simulink model "util_quat_hrn"  (R2014b)
settings: Solver=FixedStepDiscrete  StartTime=0.0  StopTime=12  FixedStep=1  RelTol=1e-3
libraries: util_quat_lib x8
settings Model: RequirementInfo={'other' './util_quat_req.html' '' 'true' ' Requirements for Quaternions' '' } %GIDa_d58dfe71_7bd5_46f6_9629_ed2cd7b47ed5  ExtModeAutoUpdateStatusClock=off  Creator=hcannon  LastModifiedBy=mstewart
settings DataIOCC: SignalLoggingSaveFormat=ModelDataLogs
settings OptimizationCC: ExpressionDepthLimit=2147483647  InitFltsAndDblsToZero=on
settings DebuggingCC: UnderspecifiedInitializationDetection=Classic  MergeDetectMultiDrivingBlocksExec=none  FcnCallInpInsideContextMsg=UseLocalSettings  StateNameClashWarn=warning  StrictBusMsg=Warning
settings SFSimCC: SimParseCustomCode=off
settings GRTTargetCC: CombineOutputUpdateFcns=off  GRTInterface=on

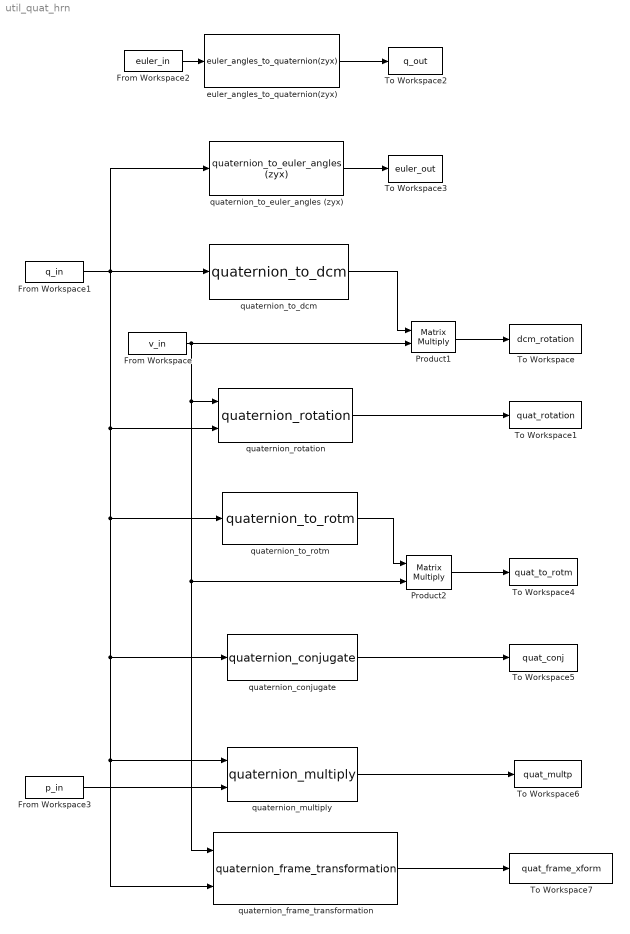
== system util_quat_hrn ==
  From Workspace : FromWorkspace  VariableName=v_in  SampleTime=0
  From Workspace1 : FromWorkspace  VariableName=q_in  SampleTime=0
  From Workspace2 : FromWorkspace  VariableName=euler_in  SampleTime=0
  From Workspace3 : FromWorkspace  VariableName=p_in  SampleTime=0
  Product1 : Product  Multiplication=Matrix(*)  RndMeth=Zero
  Product2 : Product  Multiplication=Matrix(*)  RndMeth=Zero
  To Workspace : ToWorkspace  VariableName=dcm_rotation  SampleTime=-1
  To Workspace1 : ToWorkspace  VariableName=quat_rotation  SampleTime=-1
  To Workspace2 : ToWorkspace  VariableName=q_out  SampleTime=-1
  To Workspace3 : ToWorkspace  VariableName=euler_out  SampleTime=-1
  To Workspace4 : ToWorkspace  VariableName=quat_to_rotm  SampleTime=-1
  To Workspace5 : ToWorkspace  VariableName=quat_conj  SampleTime=-1
  To Workspace6 : ToWorkspace  VariableName=quat_multp  SampleTime=-1
  To Workspace7 : ToWorkspace  VariableName=quat_frame_xform  SampleTime=-1
  euler_angles_to_quaternion(zyx) : util_quat_lib/euler_angles_to_quaternion(zyx)  SystemSampleTime=-1
  quaternion_conjugate : util_quat_lib/quaternion_conjugate  SystemSampleTime=-1
  quaternion_frame_transformation : util_quat_lib/quaternion_frame_transformation  SystemSampleTime=-1
  quaternion_multiply : util_quat_lib/quaternion_multiply  SystemSampleTime=-1
  quaternion_rotation : util_quat_lib/quaternion_rotation  SystemSampleTime=-1
  quaternion_to_dcm : util_quat_lib/quaternion_to_dcm  SystemSampleTime=-1
  quaternion_to_euler_angles (zyx) : util_quat_lib/quaternion_to_euler_angles (zyx)  SystemSampleTime=-1
  quaternion_to_rotm : util_quat_lib/quaternion_to_rotm  SystemSampleTime=-1
  wires:
  quaternion_to_dcm/1 -> Product1/1
  From Workspace1/1 -> quaternion_to_dcm/1, quaternion_to_euler_angles (zyx)/1, quaternion_rotation/2, quaternion_conjugate/1, quaternion_multiply/1, quaternion_frame_transformation/2, quaternion_to_rotm/1
  From Workspace/1 -> Product1/2, quaternion_rotation/1, Product2/2, quaternion_frame_transformation/1
  Product1/1 -> To Workspace/1
  quaternion_rotation/1 -> To Workspace1/1
  From Workspace2/1 -> euler_angles_to_quaternion(zyx)/1
  euler_angles_to_quaternion(zyx)/1 -> To Workspace2/1
  quaternion_to_euler_angles (zyx)/1 -> To Workspace3/1
  Product2/1 -> To Workspace4/1
  quaternion_to_rotm/1 -> Product2/1
  quaternion_conjugate/1 -> To Workspace5/1
  From Workspace3/1 -> quaternion_multiply/2
  quaternion_multiply/1 -> To Workspace6/1
  quaternion_frame_transformation/1 -> To Workspace7/1
